simulink model "MyClutch_RTW"  (Simulink 8.7)
settings: Solver=ode1  SolverMode=SingleTasking  StartTime=0.0  StopTime=inf  FixedStep=0.0002  RelTol=1e-3
PreLoadFcn:
  | vehicle = 'Car'; if ~length(which('cmcmd')), cmenv; end
  | MyClutch_RTW_bus
InitFcn:
  | vehicle = 'Car'; if ~length(which('cmcmd')), cmenv; end
  | MyClutch_RTW_bus
undefined symbols (not defined in the file): DiscIntNeverNeededParam
libraries: CarMaker4SL x4, simulink x1
Description:
  | CarMaker Plug-in Model Target
settings Model: Creator=ml  LastModifiedBy=IPG
settings DataIOCC: SignalLoggingSaveFormat=ModelDataLogs
settings OptimizationCC: ExpressionDepthLimit=2147483647
settings DebuggingCC: FcnCallInpInsideContextMsg=UseLocalSettings  StateNameClashWarn=warning
settings HardwareCC: TargetHWDeviceType=32-bit Generic  ProdEqTarget=off
settings RTWCC: SystemTargetFile=CarMaker.tlc  TemplateMakefile=CarMaker_unix-linux64.tmf  Description=CarMaker Plug-in Model Target
settings CodeAppCC: MaxIdLength=63
settings STFCustomTargetCC: ModelReferenceCompliant=off  GeneratePreprocessorConditionals=Disable all  MultiInstanceERTCode=on  CodeInterfacePackaging=Reusable function  CPPClassGenCompliant=on  GRTInterface=off  GenerateAllocFcn=on  SystemTargetFile=CarMaker.tlc
settings GRTTargetCC: ModelReferenceCompliant=off  ParMdlRefBuildCompliant=off  CompOptLevelCompliant=off  ConcurrentExecutionCompliant=off  CombineOutputUpdateFcns=off  MatFileLogging=off  MultiInstanceERTCode=on  CodeInterfacePackaging=Reusable function  GenerateAllocFcn=on  UseToolchainInfoCompliant=off  ExtModeMexFile=noextcomm
settings CustomProperty: DataType=string  Value=..
settings EnumStrPairs: String=Car

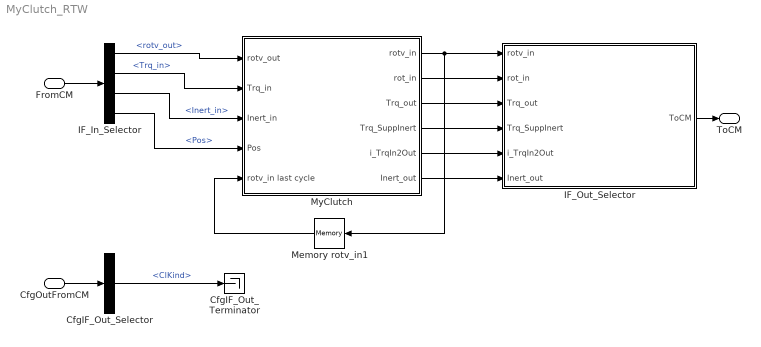
== system MyClutch_RTW ==
  FromCM : Inport  OutDataTypeStr=Bus: cmPTClutchIn
  CfgOutFromCM : Inport  Port=2  OutDataTypeStr=Bus: cmPTClutchCfgOut
  CfgIF_Out_Selector : BusSelector  OutputSignals=ClKind
  CfgIF_Out_Terminator : Terminator
  IF_In_Selector : BusSelector  OutputSignals=rotv_out,Trq_in,Inert_in,Pos
  IF_Out_Selector : Subsystem  mask(Signal Selection){}
      mask help: Signal Selection Block
      settings: OpenFcn=cmSignalSelect('SignalSelection_CB',gcb)
  Memory rotv_in1 : Memory
  MyClutch : Subsystem
  ToCM : Outport  OutDataTypeStr=Bus: cmPTClutchOut
  wires:
  FromCM/1 -> IF_In_Selector/1
  IF_Out_Selector/1(ToCM) -> ToCM/1
  CfgOutFromCM/1 -> CfgIF_Out_Selector/1
  CfgIF_Out_Selector/1 -> CfgIF_Out_Terminator/1  "<ClKind>"
  MyClutch/1(rotv_in) -> Memory rotv_in1/1, IF_Out_Selector/1(rotv_in)
  MyClutch/2(rot_in) -> IF_Out_Selector/2(rot_in)
  MyClutch/3(Trq_out) -> IF_Out_Selector/3(Trq_out)
  MyClutch/4(Trq_SuppInert) -> IF_Out_Selector/4(Trq_SuppInert)
  MyClutch/5(i_TrqIn2Out) -> IF_Out_Selector/5(i_TrqIn2Out)
  MyClutch/6(Inert_out) -> IF_Out_Selector/6(Inert_out)
  Memory rotv_in1/1 -> MyClutch/5(rotv_in last cycle)
  IF_In_Selector/1 -> MyClutch/1(rotv_out)  "<rotv_out>"
  IF_In_Selector/2 -> MyClutch/2(Trq_in)  "<Trq_in>"
  IF_In_Selector/3 -> MyClutch/3(Inert_in)  "<Inert_in>"
  IF_In_Selector/4 -> MyClutch/4(Pos)  "<Pos>"

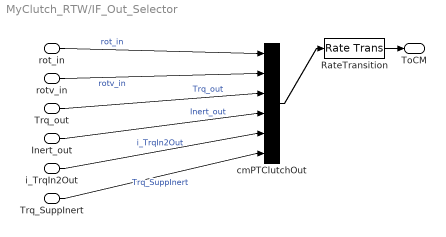
== system MyClutch_RTW/IF_Out_Selector ==
  rotv_in : Inport
  rot_in : Inport  Port=2
  Trq_out : Inport  Port=3
  Trq_SuppInert : Inport  Port=4
  i_TrqIn2Out : Inport  Port=5
  Inert_out : Inport  Port=6
  RateTransition : RateTransition  OutPortSampleTime=str2num(get_param(bdroot,'FixedStep'))
  cmPTClutchOut : BusCreator  Inputs=6
  ToCM : Outport
  wires:
  RateTransition/1 -> ToCM/1
  cmPTClutchOut/1 -> RateTransition/1
  rotv_in/1 -> cmPTClutchOut/2  "rotv_in"
  rot_in/1 -> cmPTClutchOut/1  "rot_in"
  Trq_out/1 -> cmPTClutchOut/3  "Trq_out"
  Trq_SuppInert/1 -> cmPTClutchOut/6  "Trq_SuppInert"
  i_TrqIn2Out/1 -> cmPTClutchOut/5  "i_TrqIn2Out"
  Inert_out/1 -> cmPTClutchOut/4  "Inert_out"

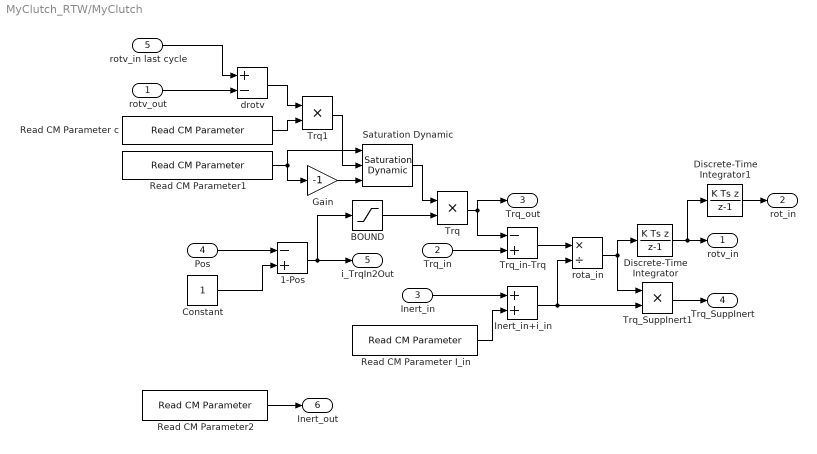
== system MyClutch_RTW/MyClutch ==
  rotv_out : Inport
  Trq_in : Inport  Port=2
  Inert_in : Inport  Port=3
  Pos : Inport  Port=4
  rotv_in last cycle : Inport  Port=5
  1-Pos : Sum  Inputs=-+
  BOUND : Saturate  UpperLimit=1  LowerLimit=0
  Constant : Constant
  Discrete-Time Integrator : DiscreteIntegrator  IntegratorMethod=Integration: Backward Euler  SampleTime=-1  ICPrevOutput=DiscIntNeverNeededParam  ICPrevScaledInput=DiscIntNeverNeededParam
  Discrete-Time Integrator1 : DiscreteIntegrator  IntegratorMethod=Integration: Backward Euler  SampleTime=-1  ICPrevOutput=DiscIntNeverNeededParam  ICPrevScaledInput=DiscIntNeverNeededParam
  Gain : Gain  Gain=-1
  Inert_in+i_in : Sum
  Read CM Parameter I_in : CarMaker4SL/Read CM Parameter  xfile=Vehicle  xkey=PowerTrain.Clutch.I_in  xnout=1  xdefaults=1e-4  xmuxed=on
  Read CM Parameter c : CarMaker4SL/Read CM Parameter  xfile=Vehicle  xkey=PowerTrain.MyClutch.c  xnout=1  xdefaults=[]  xmuxed=on
  Read CM Parameter1 : CarMaker4SL/Read CM Parameter  xfile=Vehicle  xkey=PowerTrain.Clutch.Trq_max  xnout=1  xdefaults=500  xmuxed=on
  Read CM Parameter2 : CarMaker4SL/Read CM Parameter  xfile=Vehicle  xkey=PowerTrain.Clutch.I_out  xnout=1  xdefaults=1e-4  xmuxed=on
  Saturation Dynamic : simulink/Discontinuities/Saturation Dynamic  SystemSampleTime=-1  OutMin=[]  OutMax=[]  OutDataTypeStr=Inherit: Same as second input  OutDataType=sfix(16)  OutScaling=2^-10  DoSatur=off
  Trq : Product  RndMeth=Zero
  Trq1 : Product  RndMeth=Zero
  Trq_SuppInert1 : Product  RndMeth=Zero
  Trq_in-Trq : Sum  Inputs=-+
  drotv : Sum  Inputs=+-
  rota_in : Product  Inputs=*/
  rotv_in : Outport
  rot_in : Outport  Port=2
  Trq_out : Outport  Port=3
  Trq_SuppInert : Outport  Port=4
  i_TrqIn2Out : Outport  Port=5
  Inert_out : Outport  Port=6
  wires:
  rotv_out/1 -> drotv/2
  Trq/1 -> Trq_in-Trq/1, Trq_out/1
  Trq_in/1 -> Trq_in-Trq/2
  Inert_in+i_in/1 -> rota_in/2, Trq_SuppInert1/2
  rota_in/1 -> Trq_SuppInert1/1, Discrete-Time Integrator/1
  Trq_SuppInert1/1 -> Trq_SuppInert/1
  Trq_in-Trq/1 -> rota_in/1
  rotv_in last cycle/1 -> drotv/1
  Read CM Parameter2/1 -> Inert_out/1
  Read CM Parameter c/1 -> Trq1/2
  drotv/1 -> Trq1/1
  BOUND/1 -> Trq/2
  Saturation Dynamic/1 -> Trq/1
  Read CM Parameter1/1 -> Saturation Dynamic/1, Gain/1
  Trq1/1 -> Saturation Dynamic/2
  Read CM Parameter I_in/1 -> Inert_in+i_in/2
  Inert_in/1 -> Inert_in+i_in/1
  Constant/1 -> 1-Pos/2
  Pos/1 -> 1-Pos/1
  1-Pos/1 -> BOUND/1, i_TrqIn2Out/1
  Gain/1 -> Saturation Dynamic/3
  Discrete-Time Integrator/1 -> rotv_in/1, Discrete-Time Integrator1/1
  Discrete-Time Integrator1/1 -> rot_in/1
